simulink model "Car_22_Jan_test_2012b"  (R2012b)
settings: Solver=ode5  StartTime=0.0  StopTime=inf  FixedStep=sample_time  RelTol=1e-3
InitFcn:
  | sample_time=0.005;%0.004;%0.0025;%0.02;
  | sample_time_Vicon = 0.005;
  | DeltaT = 0.02;
  | g = 9.81;
  | H0 = g%0.3165;
  | Kl = 1;
  | 
  | Q6_mass = 0.84;
  | 
  | Q6_Omega_r = 1.5; %for horizon ref
  | Q6_Zeta_r = 0.5; %for horizon ref
  | Q6_Omega_r_h = 2;%for vertical ref
  | Q6_Zeta_r_h = 2; %for vertical ref
  | 
  | 
  | Q6_Omega = 1.5; %for horizon control
  | Q6_Zeta = 0.5; %for horizon control
  | Q6_Omega_h= 2; %for vertical control
  | Q6_Zeta_h = 0.7; %for vertical control
  | 
  | 
  | Q6_acc_max = 5;%horizontal max acc
  | Q6_acc_max_h = 3;%horizontal max acc
  | 
  | omega_circle = 72*pi/180;
  | omega_h = 0.1;%Ascending speed
  | PI = pi;
  | Circle_R = 2.5;
  | MAX_Height = -2;
undefined symbols (not defined in the file or in its folder): DiscIntNeverNeededParam
libraries: X330_Control x5, dspswit3 x5, simulink x4
(part 1 of 2)
settings Model: Creator=ttcl3  LastModifiedBy=Vicon
settings SolverCC: MaxConsecutiveMinStep=auto
settings DataIOCC: SignalLoggingSaveFormat=ModelDataLogs
settings DebuggingCC: MultiTaskRateTransMsg=warning  FcnCallInpInsideContextMsg=EnableAllAsWarning
settings SFSimCC: SimParseCustomCode=off
settings CodeAppCC: CustomSymbolStrType=$N$R$M_T
settings GRTTargetCC: CombineOutputUpdateFcns=off  GRTInterface=on

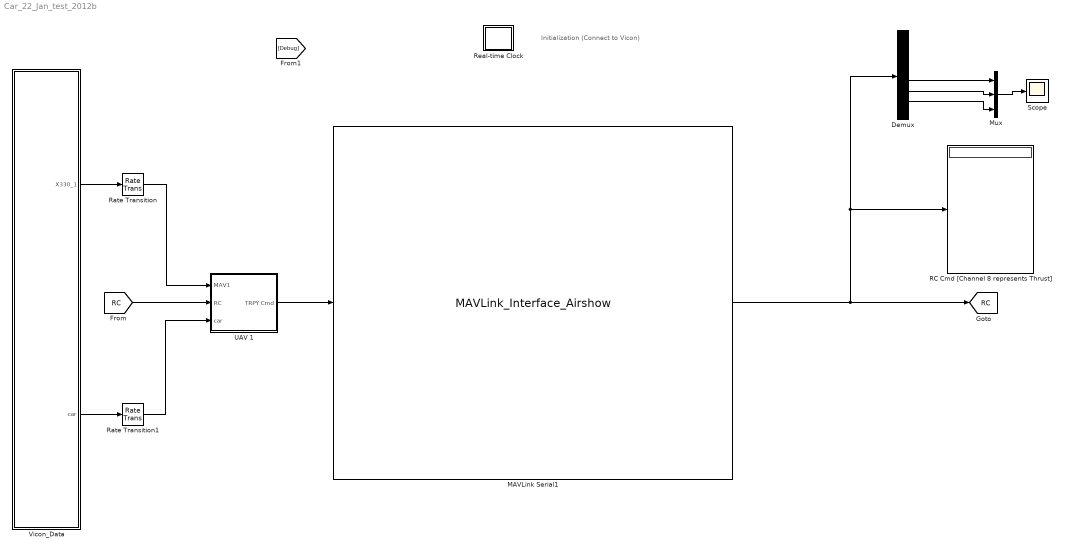
== system Car_22_Jan_test_2012b ==
  note: Initialization
      | (Connect to Vicon)
  Demux : Demux  Outputs=8
  MAVLink Serial1 : S-Function  FunctionName=MAVLink_Interface_Airshow  Parameters=COM_Port,Baud_Rate,MSG_INPUT,MSG_OUTPUT  EnableBusSupport=off  mask{COM_Port='COM5', Baud_Rate=57600, ATTITUDE_OUT=off, RC_SCALED=on, Quads_1=on, Quads_2=off, Quads_3=off, Quads_4=off, Quads_5=off, Quads_6=off}
      mask prompts: COM_Port "COM Port"; Baud_Rate "Baud Rate"; ATTITUDE_OUT "DEBUG"; RC_SCALED "RC CHANNELS SCALED"; Quads_1 "1 Quad"; Quads_2 "2 Quad"; Quads_3 "3 Quad"; Quads_4 "4 Quad"; Quads_5 "5 Quad"; Quads_6 "6 Quad"
      mask init:
      | MSG_ID_NUM_INPUT = [ uint8(221) uint8(222) uint8(223) uint8(224) uint8(225) uint8(226)];
      | MSG_ID_NAME_INPUT = [Quads_1 Quads_2 Quads_3 Quads_4 Quads_5 Quads_6];
      | 
      | MSG_ID_NUM_OUTPUT = [uint8(34) uint8(30)];
      | MSG_ID_NAME_OUTPUT = [RC_SCALED ATTITUDE_OUT ];
      | 
      | idx_input = find(MSG_ID_NAME_INPUT);
      | MSG_INPUT = MSG_ID_NUM_INPUT(idx_input);
      | 
      | idx_output = find(MSG_ID_NAME_OUTPUT);
      | MSG_OUTPUT = MSG_ID_NUM_OUTPUT(idx_output);
      mask Display:
      | % Block image
      | image(imread('10-inch Quad Heat Map.png'));
      | 
      | %Label block
      | fprintf('MAVLink Serial\n%s\n%dbps', COM_Port,  Baud_Rate)
      | 
      | 
      | %Label input ports
      | 
      | in = 1;
      | if (Quads_1 == 1)
      |     port_label('input', in, 'Quads_1');
      |     in = in + 1;
      | end
      | 
      | if (Quads_2 == 1)
      |     port_label('input', in, 'Quads_2');
      |     in = in + 1;
      | end
      | 
      | if (Quads_3 == 1)
      |     port_label('input', in, 'Quads_3');
      |     in = in + 1;
      | end
      | 
      | if (Quads_4 == 1)
      |     port_label('input', in, 'Quads_4');
      |     in = in + 1;
      | end
      | 
      | if (Quads_5 == 1)
      |     port_label('input', in, 'Quads_5');
      |     in = in + 1;
      | end
      | 
      | 
      | if (Quads_6 == 1)
      |     port_label('input', in, 'Quads_6');
      |     in = in + 1;
      | end
      | %Label output ports
      | 
      | out = 1;
      | if (RC_SCALED == 1)
      |     port_label('output', out, 'RC CMD');
      |     out = out + 1;
      | end
      | 
      | if (ATTITUDE_OUT == 1)
      |     port_label('output', out, 'DEBUG');
      |     out = out + 1;
      | end
  Mux : Mux  Inputs=3
  RC Cmd [Channel 8 represents Thrust] : Display
  Rate Transition : RateTransition  OutPortSampleTime=0.02
  Rate Transition1 : RateTransition  OutPortSampleTime=0.02
  Real-time Clock : Subsystem  mask(Real-time Clock){sample_time=0.02, tolerance=1}
      mask prompts: sample_time "Synchronize with real-time every n seconds:"; tolerance "Real-time warning tolerance (seconds):"
      mask help: Real-time Synchronization Block
      mask Help: This block synchronizes simulation time with the PC real-time clock or UNIX system clock. The first dialog entry is the period at which the clock is checked to insure real-time synchronization. The second dialog entry is the number of seconds that the simulation time must be within real-time before a warning is printed.
      mask Display: plot(0,0,100,100,[40,60,60,54,54,64,69,76,82,77,81,83,83,81,78,74,70,64,57,49,41,35,32,30,30,31,34,40,47,47,40,40],[90,90,85,85,80,79,76,87,80,70,64,57,49,41,33,28,24,22,21,23,25,31,37,46,56,65,73,78,80,85,85,90],[69,53,53],[64,50,73])
  Scope : Scope
  UAV 1 : Subsystem
  Vicon_Data : Subsystem
  tag scope: RC=global
  wires:
  [RC] -> UAV 1/2(RC)
  Vicon_Data/1(X330_1) -> Rate Transition/1
  Rate Transition/1 -> UAV 1/1(MAV1)
  UAV 1/1(TRPY Cmd) -> MAVLink Serial1/1
  Vicon_Data/2(car) -> Rate Transition1/1
  MAVLink Serial1/1 -> [RC], Demux/1, RC Cmd [Channel 8 represents Thrust]/1
  Rate Transition1/1 -> UAV 1/3(car)
  Demux/5 -> Mux/1
  Demux/6 -> Mux/2
  Demux/7 -> Mux/3
  Mux/1 -> Scope/1

== system Car_22_Jan_test_2012b/Real-time Clock ==
  Real-time Clock : S-Function  FunctionName=rtclock  Parameters=sample_time, tolerance  EnableBusSupport=off

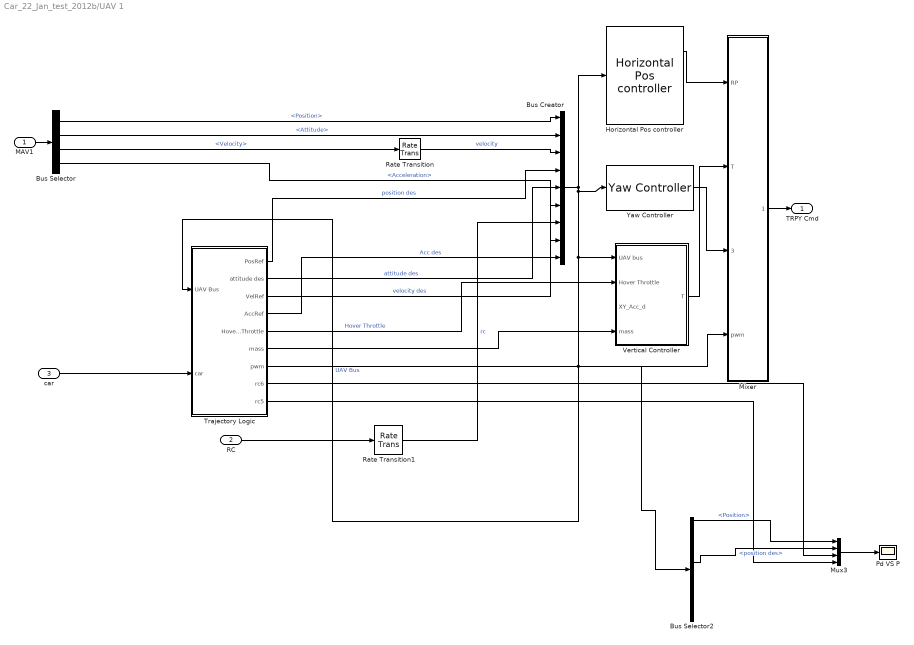
== system Car_22_Jan_test_2012b/UAV 1 ==
  MAV1 : Inport
  RC : Inport  Port=2
  car : Inport  Port=3
  Bus Creator : BusCreator  Inputs=9
  Bus Selector : BusSelector  OutputSignals=Position,Attitude,Velocity,Acceleration
  Bus Selector2 : BusSelector  OutputSignals=Position,Attitude,velocity,position des,attitude des,velocity des,rc,Acc des
  Horizontal Pos controller : X330_Control/Horizontal Pos controller  Max_RP=60  Omega=Q6_Omega  PID_i=1  Zeta=Q6_Zeta
  Mixer : Subsystem
  Mux3 : Mux
  Pd VS P : Scope
      settings: TimeRange=10  YMin=-1.5  YMax=2.25
  Rate Transition : RateTransition  OutPortSampleTime=0.02
  Rate Transition1 : RateTransition  OutPortSampleTime=0.02
  Trajectory Logic : Subsystem
  Vertical Controller : Subsystem  AncestorBlock=X330_Control/Vertical Controller  mask{Omega_h=Q6_Omega_h, Zeta_h=Q6_Zeta_h, PID_I_h=1, mass=Q6_mass}
      mask prompts: Omega_h "Omega (P Gain  = Omega^2)"; Zeta_h "Zeta (D Gain = 2*Omega*Zeta)"; PID_I_h "I Gain"
  Yaw Controller : X330_Control/Yaw Controller
  TRPY Cmd : Outport
  wires:
  Mux3/1 -> Pd VS P/1
  Bus Selector2/4 -> Mux3/2  "<position des>"
  Bus Selector2/1 -> Mux3/1  "<Position>"
  RC/1 -> Rate Transition1/1
  Trajectory Logic/4(AccRef) -> Bus Creator/9  "Acc des"
  Mixer/1(XYZ RPY) -> TRPY Cmd/1
  MAV1/1 -> Bus Selector/1
  Bus Selector/3 -> Rate Transition/1  "<Velocity>"
  Bus Selector/2 -> Bus Creator/2  "<Attitude>"
  Bus Selector/1 -> Bus Creator/1  "<Position>"
  Trajectory Logic/5(HoverThrottle) -> Vertical Controller/2(Hover Throttle)  "Hover Throttle"
  Trajectory Logic/3(VelRef) -> Bus Creator/6  "velocity des"
  Trajectory Logic/2(attitude des) -> Bus Creator/5  "attitude des"
  Trajectory Logic/1(PosRef) -> Bus Creator/4  "position des"
  Bus Selector/4 -> Bus Creator/8  "<Acceleration>"
  Vertical Controller/1(T) -> Mixer/2(T)
  Yaw Controller/1 -> Mixer/3(Yaw rate)
  Bus Creator/1 -> Yaw Controller/1, Bus Selector2/1, Trajectory Logic/1(UAV Bus), Vertical Controller/1(UAV bus), Horizontal Pos controller/1  "UAV Bus"
  Rate Transition1/1 -> Bus Creator/7  "rc"
  Rate Transition/1 -> Bus Creator/3  "velocity"
  Horizontal Pos controller/1 -> Mixer/1(RP)
  car/1 -> Trajectory Logic/2(car)
  Trajectory Logic/6(mass) -> Vertical Controller/4(mass)
  Trajectory Logic/7(pwm) -> Mixer/4(pwm)
  Trajectory Logic/8(rc6) -> Mux3/3
  Trajectory Logic/9(rc5) -> Mux3/4

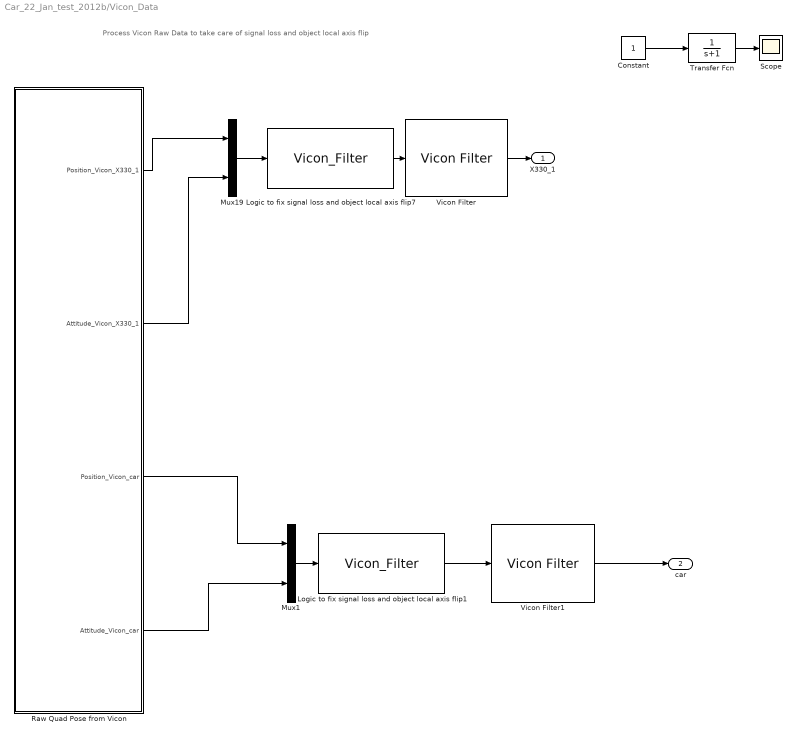
== system Car_22_Jan_test_2012b/Vicon_Data ==
  note: Process Vicon Raw Data to take care of signal loss and object local axis flip
  Constant : Constant  SampleTime=5
  Logic to fix signal loss and object local axis flip1 : M-S-Function  FunctionName=Vicon_Filter
  Logic to fix signal loss and object local axis flip7 : M-S-Function  FunctionName=Vicon_Filter
  Mux1 : Mux  Inputs=2
  Mux19 : Mux  Inputs=2
  Raw Quad Pose from Vicon : Subsystem
  Scope : Scope
      settings: SaveName=ScopeData2
  Transfer Fcn : TransferFcn  Denominator=[1 1]
  Vicon Filter : X330_Control/Vicon Filter
  Vicon Filter1 : X330_Control/Vicon Filter
  X330_1 : Outport
  car : Outport  Port=2
  wires:
  Mux19/1 -> Logic to fix signal loss and object local axis flip7/1
  Raw Quad Pose from Vicon/1(Position_Vicon_X330_1) -> Mux19/1
  Raw Quad Pose from Vicon/2(Attitude_Vicon_X330_1) -> Mux19/2
  Logic to fix signal loss and object local axis flip7/1 -> Vicon Filter/1
  Constant/1 -> Transfer Fcn/1
  Transfer Fcn/1 -> Scope/1
  Mux1/1 -> Logic to fix signal loss and object local axis flip1/1
  Logic to fix signal loss and object local axis flip1/1 -> Vicon Filter1/1
  Raw Quad Pose from Vicon/3(Position_Vicon_car) -> Mux1/1
  Raw Quad Pose from Vicon/4(Attitude_Vicon_car) -> Mux1/2
  Vicon Filter/1 -> X330_1/1
  Vicon Filter1/1 -> car/1

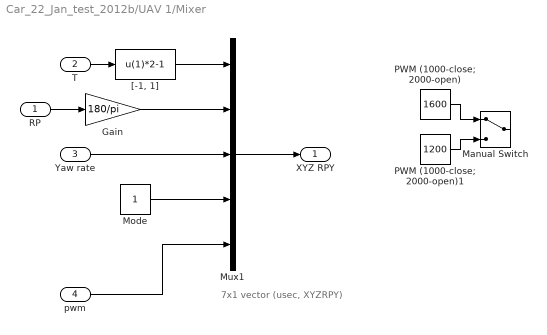
== system Car_22_Jan_test_2012b/UAV 1/Mixer ==
  note: 7x1 vector (usec, XYZRPY)
  RP : Inport
  T : Inport  Port=2
  Yaw rate : Inport  Port=3
  pwm : Inport  Port=4
  Gain : Gain  Gain=180/pi
  Manual Switch : ManualSwitch
  Mode : Constant  SampleTime=0.02
  Mux1 : Mux  Inputs=5
  PWM (1000-close; 2000-open) : Constant  Value=1600  SampleTime=0.02
  PWM (1000-close; 2000-open)1 : Constant  Value=1200  SampleTime=0.02
  "[-1, 1]" : Fcn  Expr=u(1)*2-1
  XYZ RPY : Outport
  wires:
  "[-1, 1]"/1 -> Mux1/1
  Gain/1 -> Mux1/2
  PWM (1000-close; 2000-open)1/1 -> Manual Switch/2
  PWM (1000-close; 2000-open)/1 -> Manual Switch/1
  Yaw rate/1 -> Mux1/3
  RP/1 -> Gain/1
  T/1 -> "[-1, 1]"/1
  Mux1/1 -> XYZ RPY/1
  Mode/1 -> Mux1/4
  pwm/1 -> Mux1/5

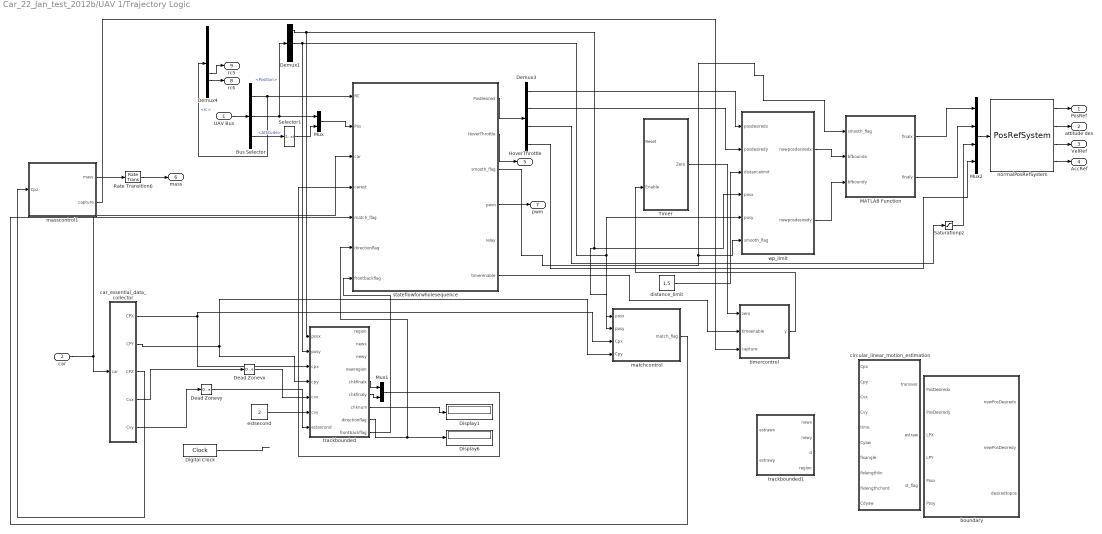
== system Car_22_Jan_test_2012b/UAV 1/Trajectory Logic ==
  UAV Bus : Inport
  car : Inport  Port=2
  Bus Selector : BusSelector  OutputSignals=rc,Position,Attitude
  Dead Zonevx : DeadZone  LowerValue=-0.1  UpperValue=0.1  SaturateOnIntegerOverflow=on
  Dead Zonevy : DeadZone  LowerValue=-0.1  UpperValue=0.1  SaturateOnIntegerOverflow=on
  Demux1 : Demux  Outputs=3
  Demux3 : Demux
  Demux4 : Demux  Outputs=8
  Digital Clock : DigitalClock  SampleTime=DeltaT
  Display1 : Display
  Display6 : Display
  MATLAB Function : MATLAB Function  TreatAsAtomicUnit=on
  Mux : Mux  Inputs=2
  Mux1 : Mux  Inputs=2
  Mux2 : Mux
  Rate Transition6 : RateTransition  OutPortSampleTime=0.02
  Saturationpz : Saturate  UpperLimit=0  LowerLimit=-2.5
  Selector1 : Selector  InputPortWidth=3  IndexOptions=Index vector (dialog)  Indices=[3]  OutputSizes=1
  Timer : Subsystem
  boundary : MATLAB Function  TreatAsAtomicUnit=on
  car_essential_data_collector : Subsystem
  circular_linear_motion_estimation : MATLAB Function  TreatAsAtomicUnit=on
  distance_limit : Constant  Value=1.5
  estsecond : Constant  Value=2
  masscontrol1 : MATLAB Function  TreatAsAtomicUnit=on
  matchcontrol : MATLAB Function  TreatAsAtomicUnit=on
  normalPosRefSystem : X330_Control/PosRefSystem  Omega_r=Q6_Omega_r  Zeta_r=Q6_Zeta_r  Acc_Max=Q6_acc_max  Omega_h_r=Q6_Omega_r_h  Zeta_h_r=Q6_Zeta_r_h  Acc_h_Max=Q6_acc_max_h
  stateflowforwholesequence : Stateflow chart  TreatAsAtomicUnit=on
  timercontrol : MATLAB Function  TreatAsAtomicUnit=on
  trackbounded : MATLAB Function  TreatAsAtomicUnit=on
  trackbounded1 : MATLAB Function  TreatAsAtomicUnit=on
  wp_limit : MATLAB Function  TreatAsAtomicUnit=on
  PosRef : Outport
  attitude des : Outport  Port=2
  VelRef : Outport  Port=3
  AccRef : Outport  Port=4
  HoverThrottle : Outport  Port=5
  mass : Outport  Port=6
  pwm : Outport  Port=7
  rc6 : Outport  Port=8
  rc5 : Outport  Port=9
  wires:
  Mux/1 -> stateflowforwholesequence/2(Pos)
  Selector1/1 -> Mux/2
  Bus Selector/3 -> Selector1/1  "<Attitude>"
  Bus Selector/2 -> Demux1/1, Mux/1  "<Position>"
  UAV Bus/1 -> Bus Selector/1
  stateflowforwholesequence/2(HoverThrottle) -> HoverThrottle/1
  Bus Selector/1 -> Demux4/1, stateflowforwholesequence/1(RC)  "<rc>"
  normalPosRefSystem/3 -> VelRef/1
  normalPosRefSystem/1 -> PosRef/1
  normalPosRefSystem/4 -> AccRef/1
  normalPosRefSystem/2 -> attitude des/1
  stateflowforwholesequence/1(PosDesired) -> Demux3/1
  Saturationpz/1 -> Mux2/3
  Mux2/1 -> normalPosRefSystem/1
  car/1 -> stateflowforwholesequence/3(car), car_essential_data_collector/1(car)
  car_essential_data_collector/1(CPX) -> trackbounded/3(cpx), matchcontrol/3(Cpx)
  car_essential_data_collector/2(CPY) -> trackbounded/4(cpy), matchcontrol/4(Cpy)
  Digital Clock/1 -> ?
  Dead Zonevx/1 -> trackbounded/5(cvx)
  Dead Zonevy/1 -> trackbounded/6(cvy)
  Demux3/1 -> wp_limit/1(posdesiredx)
  Demux3/2 -> wp_limit/2(posdesiredy)
  Demux3/3 -> Saturationpz/1
  Demux3/4 -> Mux2/4
  Demux1/1 -> matchcontrol/1(posx), wp_limit/4(posx), trackbounded/1(posx)
  Demux1/2 -> matchcontrol/2(posy), wp_limit/5(posy), trackbounded/2(posy)
  distance_limit/1 -> wp_limit/3(distancelimit)
  masscontrol1/1(mass) -> Rate Transition6/1
  stateflowforwholesequence/3(smooth_flag) -> MATLAB Function/1(smooth_flag), wp_limit/6(smooth_flag)
  car_essential_data_collector/3(CPZ) -> masscontrol1/1(Cpz)
  wp_limit/1(newposdesiredx) -> MATLAB Function/2(bfboundx)
  wp_limit/2(newposdesiredy) -> MATLAB Function/3(bfboundy)
  MATLAB Function/1(finalx) -> Mux2/1
  MATLAB Function/2(finaly) -> Mux2/2
  matchcontrol/1(match_flag) -> stateflowforwholesequence/5(match_flag)
  Rate Transition6/1 -> mass/1
  stateflowforwholesequence/4(pwm) -> pwm/1
  car_essential_data_collector/4(Cvx) -> Dead Zonevx/1
  car_essential_data_collector/5(Cvy) -> Dead Zonevy/1
  Demux4/7 -> rc6/1
  timercontrol/1(y) -> Timer/2(Enable)
  stateflowforwholesequence/6(timerenable) -> timercontrol/2(timeenable)
  Timer/1(Zero) -> timercontrol/1(zero)
  masscontrol1/2(capture) -> timercontrol/3(capture)
  Demux4/6 -> rc5/1
  estsecond/1 -> trackbounded/7(estsecond)
  trackbounded/7(chknum) -> Display1/1
  trackbounded/8(directionflag) -> stateflowforwholesequence/6(directionflag), Display6/1
  trackbounded/5(chkfinalx) -> Mux1/1
  trackbounded/6(chkfinaly) -> Mux1/2
  Mux1/1 -> stateflowforwholesequence/4(carest)
  trackbounded/9(frontbackflag) -> stateflowforwholesequence/7(frontbackflag)

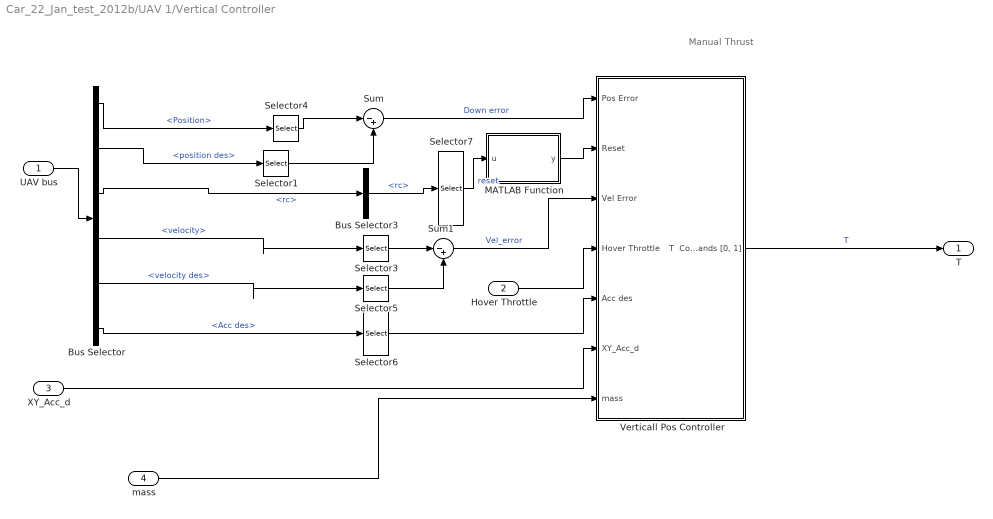
== system Car_22_Jan_test_2012b/UAV 1/Vertical Controller ==
  note: Manual Thrust
  UAV bus : Inport
  Hover Throttle : Inport  Port=2
  XY_Acc_d : Inport  Port=3
  mass : Inport  Port=4
  Bus Selector : BusSelector  OutputSignals=Position,position des,rc,velocity,velocity des,Acc des
  Bus Selector3 : BusSelector  OutputSignals=rc
  MATLAB Function : MATLAB Function  TreatAsAtomicUnit=on
  Selector{1,3..5} (4 alike) : Selector  InputPortWidth=3  IndexOptions=Index vector (dialog)  Indices=[3]  OutputSizes=1
  Selector6 : Selector  InputPortWidth=4  IndexOptions=Index vector (dialog)  Indices=[3]  OutputSizes=1
  Selector7 : Selector  InputPortWidth=8  IndexOptions=Index vector (dialog)  Indices=[7]  OutputSizes=1
  Sum : Sum  Inputs=|-+
  Sum1 : Sum  Inputs=|-+
  Verticall Pos Controller : Subsystem
  T : Outport
  wires:
  XY_Acc_d/1 -> Verticall Pos Controller/6(XY_Acc_d)
  Verticall Pos Controller/1("T  Commands [0, 1]") -> T/1  "T"
  Selector6/1 -> Verticall Pos Controller/5(Acc des)
  Bus Selector/6 -> Selector6/1  "<Acc des>"
  Hover Throttle/1 -> Verticall Pos Controller/4(Hover Throttle)
  Bus Selector/5 -> Selector5/1  "<velocity des>"
  Bus Selector/4 -> Selector3/1  "<velocity>"
  Selector5/1 -> Sum1/2
  Selector3/1 -> Sum1/1
  Sum1/1 -> Verticall Pos Controller/3(Vel Error)  "Vel_error"
  Selector7/1 -> MATLAB Function/1(u)  "reset"
  Bus Selector3/1 -> Selector7/1  "<rc>"
  Selector1/1 -> Sum/2
  Selector4/1 -> Sum/1
  Sum/1 -> Verticall Pos Controller/1(Pos Error)  "Down error"
  Bus Selector/2 -> Selector1/1  "<position des>"
  Bus Selector/1 -> Selector4/1  "<Position>"
  Bus Selector/3 -> Bus Selector3/1  "<rc>"
  UAV bus/1 -> Bus Selector/1
  mass/1 -> Verticall Pos Controller/7(mass)
  MATLAB Function/1(y) -> Verticall Pos Controller/2(Reset)

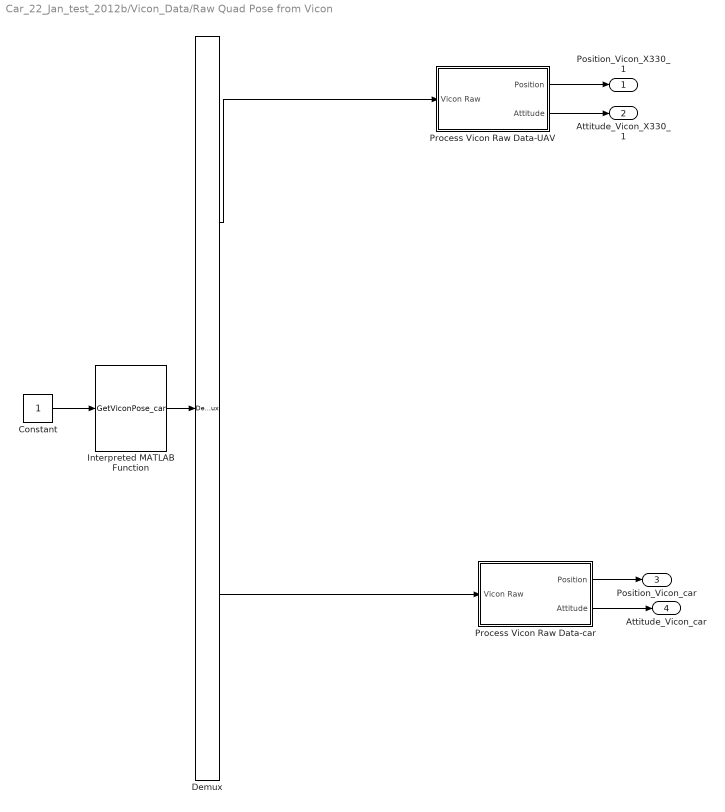
== system Car_22_Jan_test_2012b/Vicon_Data/Raw Quad Pose from Vicon ==
  Constant : Constant  SampleTime=sample_time
  Demux : Demux  Outputs=2
  Interpreted MATLAB Function : MATLABFcn  MATLABFcn=GetViconPose_car  OutputDimensions=12
  Process Vicon Raw Data-UAV : Subsystem
  Process Vicon Raw Data-car : Subsystem
  Position_Vicon_X330_1 : Outport
  Attitude_Vicon_X330_1 : Outport  Port=2
  Position_Vicon_car : Outport  Port=3
  Attitude_Vicon_car : Outport  Port=4
  wires:
  Interpreted MATLAB Function/1 -> Demux/1
  Process Vicon Raw Data-UAV/2(Attitude) -> Attitude_Vicon_X330_1/1
  Process Vicon Raw Data-UAV/1(Position) -> Position_Vicon_X330_1/1
  Demux/1 -> Process Vicon Raw Data-UAV/1(Vicon Raw)
  Constant/1 -> Interpreted MATLAB Function/1
  Process Vicon Raw Data-car/2(Attitude) -> Attitude_Vicon_car/1
  Process Vicon Raw Data-car/1(Position) -> Position_Vicon_car/1
  Demux/2 -> Process Vicon Raw Data-car/1(Vicon Raw)

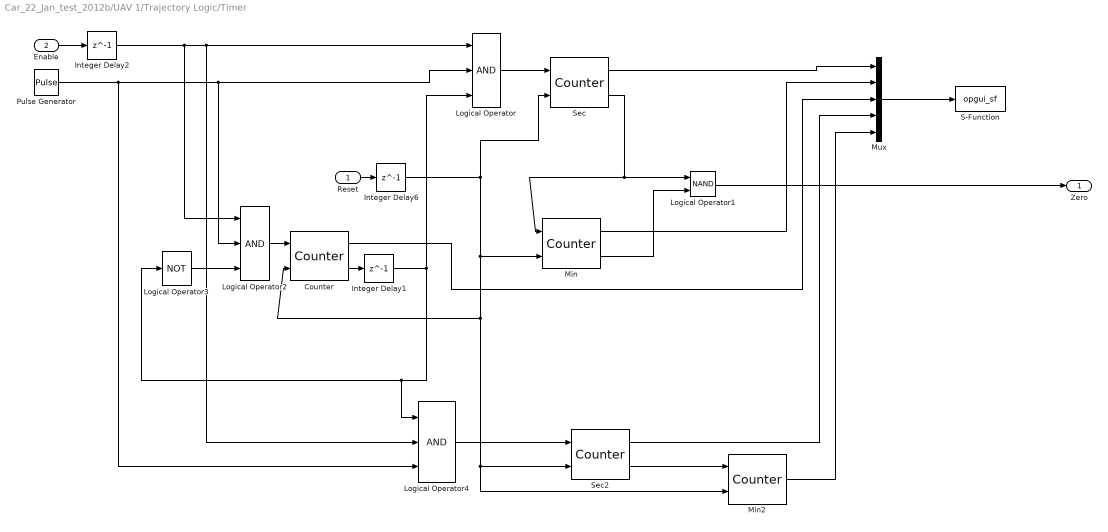
== system Car_22_Jan_test_2012b/UAV 1/Trajectory Logic/Timer ==
  Reset : Inport
  Enable : Inport  Port=2
  Counter : dspswit3/Counter  Direction=Down  CountEvent=Rising edge  CounterSize=User defined  MaxCount=4  InitialCount=4  Output=Count and Hit  HitValue=0  ResetInput=on  SamplesPerFrame=1  Ts=1  CntDtype=double  HitDtype=Boolean
  Integer Delay1 : Delay  DelayLength=1
  Integer Delay2 : Delay  DelayLength=1
  Integer Delay6 : Delay  DelayLength=1
  Logical Operator : Logic  Inputs=3  AllPortsSameDT=off  OutDataTypeStr=boolean
  Logical Operator1 : Logic  Operator=NAND  AllPortsSameDT=off  OutDataTypeStr=boolean
  Logical Operator2 : Logic  Inputs=3  AllPortsSameDT=off  OutDataTypeStr=boolean
  Logical Operator3 : Logic  Operator=NOT  Inputs=1  AllPortsSameDT=off  OutDataTypeStr=boolean
  Logical Operator4 : Logic  Inputs=3  AllPortsSameDT=off  OutDataTypeStr=boolean
  Min : dspswit3/Counter  Direction=Down  CountEvent=Rising edge  CounterSize=User defined  MaxCount=1  InitialCount=1  Output=Count and Hit  HitValue=0  ResetInput=on  SamplesPerFrame=1  Ts=1  CntDtype=double  HitDtype=Logical
  Min2 : dspswit3/Counter  Direction=Up  CountEvent=Rising edge  CounterSize=User defined  MaxCount=59  InitialCount=0  Output=Count  HitValue=0  ResetInput=on  SamplesPerFrame=1  Ts=1  CntDtype=double  HitDtype=Logical
  Mux : Mux  Inputs=5
  Pulse Generator : DiscretePulseGenerator  SampleTime=0.5
  S-Function : S-Function  FunctionName=opgui_sf  Parameters=0.5  EnableBusSupport=off
  Sec : dspswit3/Counter  Direction=Down  CountEvent=Rising edge  CounterSize=User defined  MaxCount=59  InitialCount=30  Output=Count and Hit  HitValue=0  ResetInput=on  SamplesPerFrame=1  Ts=1  CntDtype=double  HitDtype=Logical
  Sec2 : dspswit3/Counter  Direction=Up  CountEvent=Rising edge  CounterSize=User defined  MaxCount=59  InitialCount=0  Output=Count and Hit  HitValue=0  ResetInput=on  SamplesPerFrame=1  Ts=1  CntDtype=double  HitDtype=Logical
  Zero : Outport
  wires:
  Sec/2 -> Min/1, Logical Operator1/1
  Min/2 -> Logical Operator1/2
  Mux/1 -> S-Function/1
  Sec/1 -> Mux/1
  Logical Operator/1 -> Sec/1
  Counter/2 -> Integer Delay1/1
  Counter/1 -> Mux/3
  Min/1 -> Mux/2
  Logical Operator2/1 -> Counter/1
  Logical Operator3/1 -> Logical Operator2/3
  Enable/1 -> Integer Delay2/1
  Sec2/2 -> Min2/1
  Logical Operator4/1 -> Sec2/1
  Sec2/1 -> Mux/4
  Min2/1 -> Mux/5
  Integer Delay2/1 -> Logical Operator4/2, Logical Operator/1, Logical Operator2/1
  Pulse Generator/1 -> Logical Operator4/3, Logical Operator/2, Logical Operator2/2
  Reset/1 -> Integer Delay6/1
  Logical Operator1/1 -> Zero/1
  Integer Delay6/1 -> Sec/2, Counter/2, Sec2/2, Min2/2, Min/2
  Integer Delay1/1 -> Logical Operator/3, Logical Operator3/1, Logical Operator4/1

== system Car_22_Jan_test_2012b/UAV 1/Trajectory Logic/car_essential_data_collector ==
  car : Inport
  Demux : Demux  Outputs=12
  CPX : Outport
  CPY : Outport  Port=2
  CPZ : Outport  Port=3
  Cvx : Outport  Port=4
  Cvy : Outport  Port=5
  wires:
  car/1 -> Demux/1
  Demux/1 -> CPX/1
  Demux/2 -> CPY/1
  Demux/3 -> CPZ/1
  Demux/7 -> Cvx/1
  Demux/8 -> Cvy/1

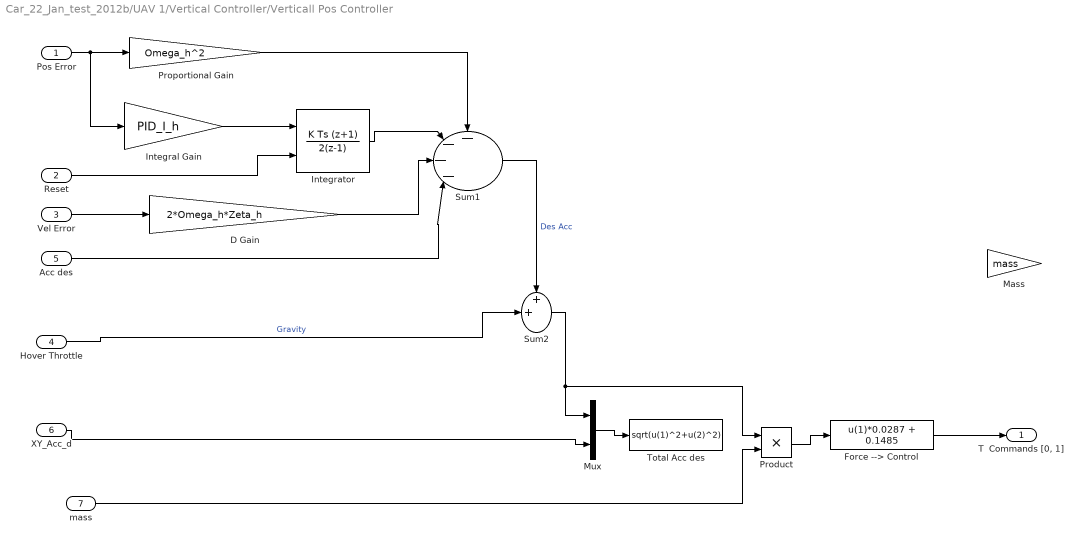
== system Car_22_Jan_test_2012b/UAV 1/Vertical Controller/Verticall Pos Controller ==
  Pos Error : Inport
  Reset : Inport  Port=2
  Vel Error : Inport  Port=3
  Hover Throttle : Inport  Port=4
  Acc des : Inport  Port=5
  XY_Acc_d : Inport  Port=6
  mass : Inport  Port=7
  D Gain : Gain  Gain=2*Omega_h*Zeta_h  OutDataTypeStr=double
  Force --> Control : Fcn  Expr=u(1)*0.0287 + 0.1485
  Integral Gain : Gain  DisableCoverage=on  Gain=PID_I_h  ParamDataTypeStr=double  OutDataTypeStr=double
  Integrator : DiscreteIntegrator  DisableCoverage=on  IntegratorMethod=Integration: Trapezoidal  ExternalReset=level  InitialConditionMode=State only (most efficient)  SampleTime=-1  OutDataTypeStr=double  UpperSaturationLimit=0.3  LowerSaturationLimit=-0.3  ICPrevOutput=DiscIntNeverNeededParam  ICPrevScaledInput=DiscIntNeverNeededParam
  Mass : Gain  DisableCoverage=on  Gain=mass  ParamDataTypeStr=double  OutDataTypeStr=double
  Mux : Mux  Inputs=2
  Product : Product  RndMeth=Zero
  Proportional Gain : Gain  DisableCoverage=on  Gain=Omega_h^2  ParamDataTypeStr=double  OutDataTypeStr=double
  Sum1 : Sum  DisableCoverage=on  Inputs=----|  AccumDataTypeStr=double  OutDataTypeStr=double  SampleTime=0.02
  Sum2 : Sum  DisableCoverage=on  Inputs=++|  AccumDataTypeStr=double  OutDataTypeStr=double  SampleTime=0.02
  Total Acc des : Fcn  Expr=sqrt(u(1)^2+u(2)^2)
  "T  Commands [0, 1]" : Outport
  wires:
  Force --> Control/1 -> "T  Commands [0, 1]"/1
  Sum2/1 -> Product/1, Mux/1
  XY_Acc_d/1 -> Mux/2
  Mux/1 -> Total Acc des/1
  Product/1 -> Force --> Control/1
  Sum1/1 -> Sum2/1  "Des Acc"
  Hover Throttle/1 -> Sum2/2  "Gravity"
  Acc des/1 -> Sum1/4
  D Gain/1 -> Sum1/3
  Vel Error/1 -> D Gain/1
  Reset/1 -> Integrator/2
  Pos Error/1 -> Integral Gain/1, Proportional Gain/1
  Proportional Gain/1 -> Sum1/1
  Integrator/1 -> Sum1/2
  Integral Gain/1 -> Integrator/1
  mass/1 -> Product/2

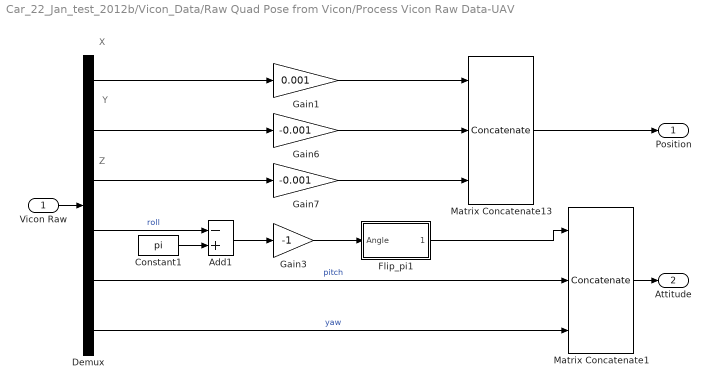
== system Car_22_Jan_test_2012b/Vicon_Data/Raw Quad Pose from Vicon/Process Vicon Raw Data-UAV ==
  note: X
  note: Y
  note: Z
  Vicon Raw : Inport
  Add1 : Sum  Inputs=-+
  Constant1 : Constant  Value=pi  OutDataTypeStr=double
  Demux : Demux  Outputs=6
  Flip_pi1 : Subsystem  mask(Flip -pi to pi){}
      mask help: Flips the inputs into the range -pi to pi
      mask Help: Flips the inputs into the range -pi to pi
      mask Display: disp('Flip_pi')
  Gain1 : Gain  Gain=0.001
  Gain3 : Gain  Gain=-1
  Gain6 : Gain  Gain=-0.001
  Gain7 : Gain  Gain=-0.001
  Matrix Concatenate1 : Concatenate  NumInputs=3  Mode=Multidimensional array
  Matrix Concatenate13 : Concatenate  NumInputs=3  Mode=Multidimensional array
  Position : Outport
  Attitude : Outport  Port=2
  wires:
  Constant1/1 -> Add1/2
  Demux/6 -> Matrix Concatenate1/3  "yaw"
  Gain1/1 -> Matrix Concatenate13/1
  Demux/1 -> Gain1/1
  Demux/2 -> Gain6/1
  Demux/3 -> Gain7/1
  Demux/4 -> Add1/1  "roll"
  Gain6/1 -> Matrix Concatenate13/2
  Gain7/1 -> Matrix Concatenate13/3
  Add1/1 -> Gain3/1
  Gain3/1 -> Flip_pi1/1(Angle)
  Demux/5 -> Matrix Concatenate1/2  "pitch"
  Flip_pi1/1(Angle_Flip) -> Matrix Concatenate1/1
  Matrix Concatenate13/1 -> Position/1
  Vicon Raw/1 -> Demux/1
  Matrix Concatenate1/1 -> Attitude/1

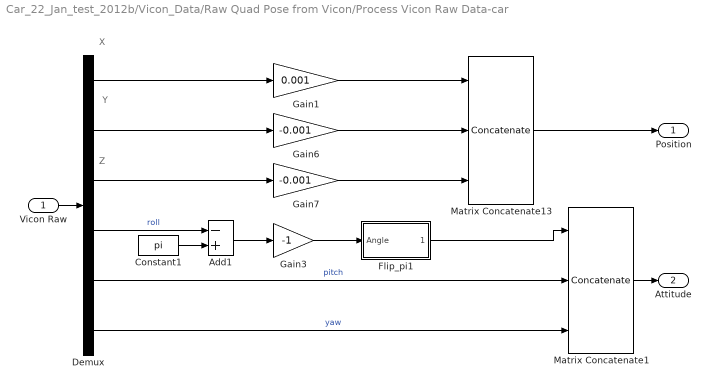
== system Car_22_Jan_test_2012b/Vicon_Data/Raw Quad Pose from Vicon/Process Vicon Raw Data-car ==
  note: X
  note: Y
  note: Z
  Vicon Raw : Inport
  Add1 : Sum  Inputs=-+
  Constant1 : Constant  Value=pi  OutDataTypeStr=double
  Demux : Demux  Outputs=6
  Flip_pi1 : Subsystem  mask(Flip -pi to pi){}
      mask help: Flips the inputs into the range -pi to pi
      mask Help: Flips the inputs into the range -pi to pi
      mask Display: disp('Flip_pi')
  Gain1 : Gain  Gain=0.001
  Gain3 : Gain  Gain=-1
  Gain6 : Gain  Gain=-0.001
  Gain7 : Gain  Gain=-0.001
  Matrix Concatenate1 : Concatenate  NumInputs=3  Mode=Multidimensional array
  Matrix Concatenate13 : Concatenate  NumInputs=3  Mode=Multidimensional array
  Position : Outport
  Attitude : Outport  Port=2
  wires:
  Constant1/1 -> Add1/2
  Demux/6 -> Matrix Concatenate1/3  "yaw"
  Gain1/1 -> Matrix Concatenate13/1
  Demux/1 -> Gain1/1
  Demux/2 -> Gain6/1
  Demux/3 -> Gain7/1
  Demux/4 -> Add1/1  "roll"
  Gain6/1 -> Matrix Concatenate13/2
  Gain7/1 -> Matrix Concatenate13/3
  Add1/1 -> Gain3/1
  Gain3/1 -> Flip_pi1/1(Angle)
  Demux/5 -> Matrix Concatenate1/2  "pitch"
  Flip_pi1/1(Angle_Flip) -> Matrix Concatenate1/1
  Matrix Concatenate13/1 -> Position/1
  Vicon Raw/1 -> Demux/1
  Matrix Concatenate1/1 -> Attitude/1

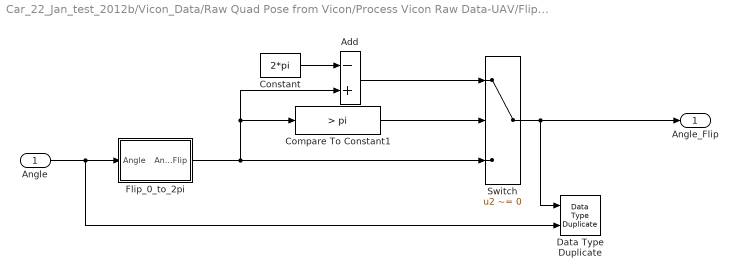
== system Car_22_Jan_test_2012b/Vicon_Data/Raw Quad Pose from Vicon/Process Vicon Raw Data-UAV/Flip_pi1 ==
  Angle : Inport
  Add : Sum  Inputs=-+
  Compare To Constant1 : simulink/Logic and Bit Operations/Compare To Constant  relop=>  const=pi  OutDataTypeStr=uint8  ZeroCross=off
  Constant : Constant  Value=2*pi
  Data Type Duplicate : DataTypeDuplicate
  Flip_0_to_2pi : Subsystem  mask(Flip zero to 2pi){}
      mask help: Flips the inputs into the range zero to +2pi
      mask Help: Flips the inputs into the range zero to +2pi
      mask Display: disp('Flip_0_2pi')
  Switch : Switch  Criteria=u2 ~= 0
  Angle_Flip : Outport
  wires:
  Switch/1 -> Data Type Duplicate/1, Angle_Flip/1
  Add/1 -> Switch/1
  Constant/1 -> Add/1
  Compare To Constant1/1 -> Switch/2
  Flip_0_to_2pi/1(Angle_Flip) -> Add/2, Compare To Constant1/1, Switch/3
  Angle/1 -> Data Type Duplicate/2, Flip_0_to_2pi/1(Angle)

== system Car_22_Jan_test_2012b/Vicon_Data/Raw Quad Pose from Vicon/Process Vicon Raw Data-car/Flip_pi1 ==
  Angle : Inport
  Add : Sum  Inputs=-+
  Compare To Constant1 : simulink/Logic and Bit Operations/Compare To Constant  relop=>  const=pi  OutDataTypeStr=uint8  ZeroCross=off
  Constant : Constant  Value=2*pi
  Data Type Duplicate : DataTypeDuplicate
  Flip_0_to_2pi : Subsystem  mask(Flip zero to 2pi){}
      mask help: Flips the inputs into the range zero to +2pi
      mask Help: Flips the inputs into the range zero to +2pi
      mask Display: disp('Flip_0_2pi')
  Switch : Switch  Criteria=u2 ~= 0
  Angle_Flip : Outport
  wires:
  Switch/1 -> Data Type Duplicate/1, Angle_Flip/1
  Add/1 -> Switch/1
  Constant/1 -> Add/1
  Compare To Constant1/1 -> Switch/2
  Flip_0_to_2pi/1(Angle_Flip) -> Add/2, Compare To Constant1/1, Switch/3
  Angle/1 -> Data Type Duplicate/2, Flip_0_to_2pi/1(Angle)

== system Car_22_Jan_test_2012b/Vicon_Data/Raw Quad Pose from Vicon/Process Vicon Raw Data-UAV/Flip_pi1/Flip_0_to_2pi ==
  Angle : Inport
  Add : Sum
  Compare To Constant1 : simulink/Logic and Bit Operations/Compare To Constant  relop=<  const=0  OutDataTypeStr=uint8  ZeroCross=off
  Constant : Constant  Value=2*pi
  Data Type Duplicate : DataTypeDuplicate
  Flip_2pi : Subsystem  mask(Flip -2pi to 2pi){}
      mask help: Flips the inputs into the range -2pi to +2pi
      mask Help: Flips the inputs into the range -2pi to +2pi
      mask Display: disp('Flip_2pi')
  Switch : Switch  Criteria=u2 ~= 0
  Angle_Flip : Outport
  wires:
  Switch/1 -> Data Type Duplicate/1, Angle_Flip/1
  Angle/1 -> Data Type Duplicate/2, Flip_2pi/1(Angle)
  Add/1 -> Switch/1
  Constant/1 -> Add/1
  Compare To Constant1/1 -> Switch/2
  Flip_2pi/1(Angle_Flip) -> Switch/3, Add/2, Compare To Constant1/1

== system Car_22_Jan_test_2012b/Vicon_Data/Raw Quad Pose from Vicon/Process Vicon Raw Data-car/Flip_pi1/Flip_0_to_2pi ==
  Angle : Inport
  Add : Sum
  Compare To Constant1 : simulink/Logic and Bit Operations/Compare To Constant  relop=<  const=0  OutDataTypeStr=uint8  ZeroCross=off
  Constant : Constant  Value=2*pi
  Data Type Duplicate : DataTypeDuplicate
  Flip_2pi : Subsystem  mask(Flip -2pi to 2pi){}
      mask help: Flips the inputs into the range -2pi to +2pi
      mask Help: Flips the inputs into the range -2pi to +2pi
      mask Display: disp('Flip_2pi')
  Switch : Switch  Criteria=u2 ~= 0
  Angle_Flip : Outport
  wires:
  Switch/1 -> Data Type Duplicate/1, Angle_Flip/1
  Angle/1 -> Data Type Duplicate/2, Flip_2pi/1(Angle)
  Add/1 -> Switch/1
  Constant/1 -> Add/1
  Compare To Constant1/1 -> Switch/2
  Flip_2pi/1(Angle_Flip) -> Switch/3, Add/2, Compare To Constant1/1

== system Car_22_Jan_test_2012b/Vicon_Data/Raw Quad Pose from Vicon/Process Vicon Raw Data-UAV/Flip_pi1/Flip_0_to_2pi/Flip_2pi ==
  Angle : Inport
  Bias : Bias  Bias=-2*pi
  Constant : Constant  Value=2*pi
  Data Type Duplicate : DataTypeDuplicate
  Modulo : Math  Operator=mod  SaturateOnIntegerOverflow=on
  Sign1 : Signum
  Switch : Switch
  Angle_Flip : Outport
  wires:
  Switch/1 -> Data Type Duplicate/2, Angle_Flip/1
  Bias/1 -> Switch/3
  Sign1/1 -> Switch/2
  Modulo/1 -> Switch/1, Bias/1
  Constant/1 -> Modulo/2
  Angle/1 -> Data Type Duplicate/1, Sign1/1, Modulo/1

== system Car_22_Jan_test_2012b/Vicon_Data/Raw Quad Pose from Vicon/Process Vicon Raw Data-car/Flip_pi1/Flip_0_to_2pi/Flip_2pi ==
  Angle : Inport
  Bias : Bias  Bias=-2*pi
  Constant : Constant  Value=2*pi
  Data Type Duplicate : DataTypeDuplicate
  Modulo : Math  Operator=mod  SaturateOnIntegerOverflow=on
  Sign1 : Signum
  Switch : Switch
  Angle_Flip : Outport
  wires:
  Switch/1 -> Data Type Duplicate/2, Angle_Flip/1
  Bias/1 -> Switch/3
  Sign1/1 -> Switch/2
  Modulo/1 -> Switch/1, Bias/1
  Constant/1 -> Modulo/2
  Angle/1 -> Data Type Duplicate/1, Sign1/1, Modulo/1

== matlab function Car_22_Jan_test_2012b/UAV 1/Trajectory Logic/circular_linear_motion_estimation ==
  data: Cpx input; Cpy input; Cvx input; Cvy input; transvec output; estraw output; st_flag output; time input; Cyaw input; fixangle input; fixlengthlin input; fixlengthchord input; Cdyaw input
function [transvec,estraw,st_flag] = fcn(Cpx,Cpy,Cvx,Cvy,time,Cyaw,fixangle,fixlengthlin,fixlengthchord,Cdyaw)
if(Cvx == 0 && Cvy == 0)
    st_flag = 1;
else 
    st_flag = 0;
end
%%%%%%%%%%%%%%%%%%%%%%circular estimation%%%%%%%%%%%%%%%%%%%%%%%%%%%%
%vxyM = sqrt((Cvx)^2 + (Cvy)^2); %resultant vector vxy
if(st_flag == 0)
    
        angleOmega = Cyaw + 0.5 * fixangle * pi / 180; %angleOmega(radian): between vx and L
        zero_chk = 1;
else
    
      angleOmega = 0;  
      zero_chk = 0;
end
if(Cdyaw ~= 0) %use dyaw to select circular or linear estimation
%r = vxyM / abs(Cdyaw);
%Chord = 2 * r * sin(fixangle * pi / 360); %%%%%chord sometime will go to
%very large value, will disable this parameter soon
transveccir = [fixlengthchord * cos(angleOmega)*zero_chk  fixlengthchord * sin(angleOmega) * zero_chk];
transveclin = [0 0];
else
%%%%%%%%%%%%%%%%%%%%%%%%linear estimation%%%%%%%%%%%%%%%%%%%%%%%%%%%%%%
transveclin = [fixlengthlin * cos(Cyaw * pi / 180)*zero_chk fixlengthlin * sin(Cyaw * pi / 180)*zero_chk];
transveccir = [0 0];
%Chord = 0;
end
if(time<2)       %%%%%%%%%%%%%%%%%avoid noise when initializing the program in first 2 seconds
    transvec = [0 0];
else
transvec = transveccir + transveclin;
end

C2dvec = [Cpx Cpy];
estraw = C2dvec + transvec;

== matlab function Car_22_Jan_test_2012b/UAV 1/Trajectory Logic/wp_limit ==
  data: posdesiredx input; posdesiredy input; distancelimit input; posx input; posy input; newposdesiredx output; newposdesiredy output; smooth_flag input
function [newposdesiredx,newposdesiredy] = fcn(posdesiredx,posdesiredy,distancelimit,posx,posy,smooth_flag)
%#codegen
w = atan2((posdesiredx-posx),(posdesiredy-posy));
desiredtopos = sqrt((posdesiredy-posy)^2+(posdesiredx-posx)^2);
if(smooth_flag == 1)
    newposdesiredx = posdesiredx;
    newposdesiredy = posdesiredy;
    %newposdesiredx = posx + smoothdistancelimit*sin(w);
    %newposdesiredy = posy + smoothdistancelimit*cos(w);
else
if(desiredtopos <= distancelimit)
    newposdesiredx = posdesiredx;
    newposdesiredy = posdesiredy;
else
    newposdesiredx = posx + distancelimit*sin(w);
    newposdesiredy = posy + distancelimit*cos(w);
end
end

== matlab function Car_22_Jan_test_2012b/UAV 1/Trajectory Logic/trackbounded1 ==
  data: newx output; newy output; estrawx input; estrawy input; d output; region output
function [newx,newy,d,region]  = fcn(estrawx,estrawy)
%#codegen
%cp = [cpy,cpx,0];
cpest = [estrawy, estrawx,0];
%%database of check points
chk0x = -0.4383;
chk0y = -0.9285;
chk1x = 1.047;
chk1y = -0.9693;
chk2x = 1.396;
chk2y = 0.4535;
chk3x = 1.382;
chk3y = 1.505;
chk4x = 1.042;
chk4y = 1.925;
chk5x = 0.3708;
chk5y = 1.821;
%%chk5x = ;
%%chk....
chk0 = [chk0y,chk0x,0];
chk1 = [chk1y,chk1x,0];
chk2 = [chk2y,chk2x,0];
chk3 = [chk3y,chk3x,0];
chk4 = [chk4y,chk4x,0];
chk5 = [chk5y,chk5x,0];
%%%%%%%%%%%%%%%%%%%%%%%%%%%%%%%%%%%%%%%%%%%%%%%%%%%%%%%%%%%%%%%%%%%%%%%%%%%%%%%%%%%%%%region selector
if(estrawx>2 && estrawx<=3 && estrawy>-3 && estrawy<=-2)
    region = 0;
elseif(estrawx>2 && estrawx<=3 && estrawy>-2 && estrawy<=-1 )
    region = 1;
elseif(estrawx>2 && estrawx<=3 && estrawy>-1 && estrawy<=0 )
    region = 2;
elseif(estrawx>2 && estrawx<=3 && estrawy>0 && estrawy<=1 )
    region = 3;
elseif(estrawx>2 && estrawx<=3 && estrawy>1 && estrawy<=2)
    region = 4;
elseif(estrawx>2 && estrawx<=3 && estrawy>2 && estrawy<=3)
    region = 5;
elseif(estrawx>1 && estrawx<=2 && estrawy>-3 && estrawy<=-2)
    region = 6;
elseif(estrawx>1 && estrawx<=2 && estrawy>-2 && estrawy<=-1)
    region = 7;
elseif(estrawx>1 && estrawx<=2 && estrawy>-1 && estrawy<=0)
    region = 8;
elseif(estrawx>1 && estrawx<=2 && estrawy>0 && estrawy<=1)
    region = 9;
elseif(estrawx>1 && estrawx<=2 && estrawy>1 && estrawy<=2)
    region = 10;
elseif(estrawx>1 && estrawx<=2 && estrawy>2 && estrawy<=3)
    region = 11;
elseif(estrawx>0 && estrawx<=1 && estrawy>-3 && estrawy<=-2)
    region = 12;
elseif(estrawx>0 && estrawx<=1 && estrawy>-2 && estrawy<=-1)
    region = 13;
elseif(estrawx>0 && estrawx<=1 && estrawy>-1 && estrawy<=0)
    region = 14;
elseif(estrawx>0 && estrawx<=1 && estrawy>0 && estrawy<=1)
    region = 15;
elseif(estrawx>0 && estrawx<=1 && estrawy>1 && estrawy<=2)
    region = 16;
elseif(estrawx>0 && estrawx<=1 && estrawy>2 && estrawy<=3)
    region = 17;
elseif(estrawx>-1 && estrawx<=0 && estrawy>-3 && estrawy<=-2)
    region = 18;
elseif(estrawx>-1 && estrawx<=0 && estrawy>-2 && estrawy<=-1)
    region = 19;
elseif(estrawx>-1 && estrawx<=0 && estrawy>-1 && estrawy<=0)
    region = 20;
elseif(estrawx>-1 && estrawx<=0 && estrawy>0 && estrawy<=1)
    region = 21;
elseif(estrawx>-1 && estrawx<=0 && estrawy>1 && estrawy<=2)
    region = 22;
elseif(estrawx>-1 && estrawx<=0 && estrawy>2 && estrawy<=3)
    region = 23;
elseif(estrawx>-2 && estrawx<=-1 && estrawy>-3 && estrawy<=-2)
    region = 24;
elseif(estrawx>-2 && estrawx<=-1 && estrawy>-2 && estrawy<=-1)
    region = 25;
elseif(estrawx>-2 && estrawx<=-1 && estrawy>-1 && estrawy<=0)
    region = 26;
elseif(estrawx>-2 && estrawx<=-1 && estrawy>0 && estrawy<=1)
    region = 27;
elseif(estrawx>-2 && estrawx<=-1 && estrawy>1 && estrawy<=2)
    region = 28;
elseif(estrawx>-2 && estrawx<=-1 && estrawy>2 && estrawy<=3)
    region = 29;
elseif(estrawx>-3 && estrawx<=-2 && estrawy>-3 && estrawy<=-2)
    region = 30;
elseif(estrawx>-3 && estrawx<=-2 && estrawy>-2 && estrawy<=-1)
    region = 31;
elseif(estrawx>-3 && estrawx<=-2 && estrawy>-1 && estrawy<=0)
    region = 32;
elseif(estrawx>-3 && estrawx<=-2 && estrawy>0 && estrawy<=1)
    region = 33;
elseif(estrawx>-3 && estrawx<=-2 && estrawy>1 && estrawy<=2)
    region = 34;
elseif(estrawx>-3 && estrawx<=-2 && estrawy>2 && estrawy<=3)
    region = 35;
else
    region = -1;
end
%%%%%%%%%%%%%%%%%%%%%%%%%%%%%%%%%%%%%%%%%%%%%%%%%%%%%%%%%%%%%%%%%%%%%%%%%%%%%%%%%%%%%%%%%%%%%%%%%%
if(region == 20 || region==19||region==13||region==14||region==7||region==21||region==6||region==12||region==18||region==24||region==25||region==26||region==27)
    %%%%%%%%%%%%%%%%calculate point to line distance%%%%%%%%%%%
    a = chk1 - chk0;
    b = cpest - chk0;
    d = norm(cross(a,b)) / norm(a);
    angle = atan2((chk1x-chk0x),(chk1y-chk0y));
    samplex = chk0x;
    sampley = chk0y;
    samplefinalx = chk1x;
    samplefinaly = chk1y;
    zero = 1;
elseif(region == 2||region==1||region==0||region==8)
    a = chk2 - chk1;
    b = cpest - chk1;
    d = norm(cross(a,b)) / norm(a);
    angle = atan2((chk2x-chk1x),(chk2y-chk1y));
    zero = 1;
    samplex = chk1x;
    sampley = chk1y;
    samplefinalx = chk2x;
    samplefinaly = chk2y;
elseif(region == 3||region==9||region==15)
    a = chk3 - chk2;
    b = cpest - chk2;
    d = norm(cross(a,b)) / norm(a);
    angle = atan2((chk3x-chk2x),(chk3y-chk2y));
    zero = 1;
    samplex = chk2x;
    sampley = chk2y;
    samplefinalx = chk3x;
    samplefinaly = chk3y;
elseif(region == 5||region==5||region==10||region==11)
    a = chk4 - chk3;
    b = cpest - chk3;
    d = norm(cross(a,b)) / norm(a);
    angle = atan2((chk4x-chk3x),(chk4y-chk3y));
    zero = 1;  
    samplex = chk3x;
    sampley = chk3y;
    samplefinalx = chk4x;
    samplefinaly = chk4y;
elseif(region == 16||region==17||region==22||region==23||region==28||region==29||region==34||region==35)
    a = chk5 - chk4;
    b = cpest - chk4;
    d = norm(cross(a,b)) / norm(a);
    angle = atan2((chk5x-chk4x),(chk5y-chk4y));
    zero = 1;
     samplex = chk4x;
    sampley = chk4y;
    samplefinalx = chk5x;
    samplefinaly = chk5y;

else
    a = -1;
    b = -1;
    d = -1;
    angle = -1;%%% i know this is not correct i will add one more zero coefficient to cancel this case
    zero = 0;
    samplex = 0;
    sampley = 0;
    samplefinalx = 0;
    samplefinaly = 0;
end
%%%%%%%%%%%%%%%%%%%%%%%%%%%%%%%%%%%%%%%%%%%%%%%%%%%%%%%%%%%%%%%%%%%%%%%%%%%%%%%%%%%%%%%%%%%%%%%%%%
%%calculate project point on the check point line
if(region == -1)%%if out of boundary none of the region match
        newy = 0;
        newx = 0;
else   %%match the region

distance = sqrt((samplefinalx-estrawx)^2+(samplefinaly-estrawy)^2); 
%if(distance > 1)
    %newx = samplefinalx;
   % newy = samplefinaly;
%else
      if(d<0.75)%%test the boundary width normal case if less than 0.75 m
    newx = estrawx;
    newy = estrawy;
      else%% out of boundary
        if(angle == 0 ||angle == 180)
            newx  = samplex;
            newy = estrawy;
        elseif(angle == 90 || angle == 270)
            newx = estrawx;
            newy = sampley;
        else
         kk = -1/(tan(angle));
         m = estrawx - kk*estrawy ;
         k = tan(angle);
         newy = (samplex - k*sampley - m)/(kk - k);
         newx = kk*newy + m;
        end
      end
%end
end

== matlab function Car_22_Jan_test_2012b/UAV 1/Trajectory Logic/boundary ==
  data: PosDesiredx input; newPosDesiredx output; PosDesiredy input; LPX input; LPY input; Posx input; Posy input; newPosDesiredy output; desiredtopos output
function [newPosDesiredx, newPosDesiredy,desiredtopos] = fcn(PosDesiredx,PosDesiredy, LPX,LPY,Posx,Posy)

UAVreal = [Posy, Posx,0];
UAVdesired = [PosDesiredy, PosDesiredx,0];
LA = [LPY, LPX,0];
r = 1.2;%%%%%landing_area circle radius
%%%%%%%%%%%%%%%%calculate point to line distance%%%%%%%%%%%
if(PosDesiredx == Posx && PosDesiredy == Posy)
    d = 1.3; %%%%%%%%%%%whatever value larger than 1.2, just for if this is not a line but a point
else
    a = UAVdesired - UAVreal;
    b = LA - UAVreal;
    d = norm(cross(a,b)) / norm(a);
end
%%%%%%%%%%%%%%%%%%%%%%%%%%%%%%%%%%%%%%%%%%%%%%%%%%%%%%%%%%
k = (PosDesiredx-Posx)/(PosDesiredy-Posy);
m = -k*PosDesiredy + PosDesiredx - LPX;
desiredtopos = sqrt((PosDesiredy-Posy)^2+(PosDesiredx-Posx)^2);
w = 0;
angleLAtoPos=atan2((Posx-LPX),(Posy-LPY));
if((Posx-LPX)^2+(Posy-LPY)^2<=r^2)%%%uav inside the circle already
    newPosDesiredx = LPX + r*cos(angleLAtoPos);
    newPosDesiredy = LPY + r*sin(angleLAtoPos);
else%%%%%%%uav outside the circle
if(d>=r)%%outside or tangent with circle
    n = 0;
    w = 0;
    zerochk = 0;
    wperpendicular = (w + 0.5 * pi)*zerochk;
    intersecty1 = Posy;
    intersecty2 = Posy;
    intersectx1 = Posx;
    intersectx2 = Posx;
    intersec1topos = sqrt((intersecty1-Posy)^2 + (intersectx1-Posx)^2);
    intersec2topos = sqrt((intersecty2-Posy)^2 + (intersectx2-Posx)^2);
    newPosDesiredy = PosDesiredy;
    newPosDesiredx = PosDesiredx;
else 
    n = sqrt(4*(LPY - k*m)^2 - 4*(k^2+1)*(LPY^2 + m^2 - r^2));
    intersecty1 = (2*(LPY - k*m)+n)/(2*(k^2+1));
    intersecty2 = (2*(LPY - k*m)-n)/(2*(k^2+1));
    intersectx1 = k*(intersecty1 - PosDesiredy)+PosDesiredx;
    intersectx2 = k*(intersecty2 - PosDesiredy)+PosDesiredx;
    intersec1topos = sqrt((intersecty1-Posy)^2 + (intersectx1-Posx)^2);
    intersec2topos = sqrt((intersecty2-Posy)^2 + (intersectx2-Posx)^2);
    if(intersec1topos<intersec2topos)
        w = atan2((LPX-intersectx1),(LPY-intersecty1));
    else
        w = atan2((LPX-intersectx2),(LPY-intersecty2));
    end
        if(desiredtopos<=intersec1topos && desiredtopos<=intersec2topos)
            newPosDesiredx = PosDesiredx;
            newPosDesiredy = PosDesiredy;
            zerochk = 0;
            wperpendicular = (w + 0.5 * pi)*zerochk;
        elseif(desiredtopos<=intersec1topos && desiredtopos>intersec2topos)
            newPosDesiredx = intersectx2;
            newPosDesiredy = intersecty2;
            zerochk = 0;
            wperpendicular = (w + 0.5 * pi)*zerochk;
        elseif(desiredtopos>intersec1topos && desiredtopos<=intersec2topos)  
            newPosDesiredx = intersectx1;
            newPosDesiredy = intersecty1;
            zerochk = 0;
            wperpendicular = (w + 0.5 * pi)*zerochk;
        else
            zerochk = 1;
            wperpendicular = (w + 0.5 * pi)*zerochk;
            if(intersec1topos<intersec2topos)
            newPosDesiredx = 0.5*cos(wperpendicular) + intersectx1;
            newPosDesiredy = 0.5*sin(wperpendicular) + intersecty1;
            else
            newPosDesiredx = 0.5*cos(wperpendicular) + intersectx2;
            newPosDesiredy = 0.5*sin(wperpendicular) + intersecty2;  
            end
            
        end
    
end 
end

== matlab function Car_22_Jan_test_2012b/UAV 1/Trajectory Logic/matchcontrol ==
  data: match_flag output; posx input; posy input; Cpx input; Cpy input
function match_flag  = fcn(posx,posy,Cpx,Cpy)
%#codegen
if(abs(Cpx-posx)+abs(Cpy-posy)<0.3)
    match_flag = 1;
else
    match_flag = 0;
end

== matlab function Car_22_Jan_test_2012b/UAV 1/Trajectory Logic/masscontrol1 ==
  data: mass output; Cpz input; capture output
function [mass,capture]  = fcn(Cpz)
%#codegen

if( Cpz <-0.1)%match_flag==1 && Cpz<=-0.07 &&
    mass = 1.2;
    capture = 0;
else
    mass = 0.84;
    capture = 1;
    
end

== matlab function Car_22_Jan_test_2012b/UAV 1/Trajectory Logic/MATLAB Function ==
  data: smooth_flag input; bfboundx input; finalx output; finaly output; bfboundy input
function [finalx,finaly] = fcn(smooth_flag,bfboundx,bfboundy)
%#codegen
if(smooth_flag == 1)
    finalx = bfboundx;
    finaly = bfboundy;
else
    if(bfboundx >= 2.489)
        finalx = 2.489;
    elseif(bfboundx <= -2.83)
        finalx = -2.83;
    else
        finalx = bfboundx;
    end
     if(bfboundy >= 3)
        finaly = 3;
    elseif(bfboundy <= -2.345)
        finaly = -2.345;
    else
        finaly = bfboundy;
     end
end

== matlab function Car_22_Jan_test_2012b/UAV 1/Trajectory Logic/timercontrol ==
  data: zero input; y output; timeenable input; capture input
function y = fcn(zero,timeenable,capture)
%#codegen
if(zero == 0||capture ==0||timeenable==0)
    y = 0;
else
   y = 1; 
end

== stateflow chart Car_22_Jan_test_2012b/UAV 1/Trajectory Logic/stateflowforwholesequence ==
  state Airborne1
    state capturing_sequence
      state caputuring_test1
        en: PosDesired = Pos; PosDesired[2] = -1.2;smooth_flag = 1;timerenable = 0;
      state capturing_sequence1
        state capturing_sequence2
          state normal_capturing1
            en: PosDesired[0] = carest[0] ; PosDesired[1] = carest[1] ; PosDesired[2] = -0.5;pwm = 1650;
          state normal_capturing3
            du: PosDesired[0] = car[0] ; PosDesired[1] = car[1]; PosDesired[2] = -0.5;pwm = 1250;
          state normal_capturing2
            du: PosDesired[0] = car[0] ; PosDesired[1] = car[1]; PosDesired[2] = -0.5;pwm = 1250;
          state match_chk
            state caputuring_test1
              en:PosDesired = Pos;PosDesired[2] = -1.2;
            state caputuring_test2
              en: PosDesired[0] = 0.15*(0-car[0])/abs(0-car[0]);
              PosDesired[1] = 0.15*(0-car[1])/abs(0-car[1]);
            state caputuring_test
              en: PosDesired[2] = -0.5;
            (default) -> (junction 60) : {PosDesired = Pos;pwm = 1450;PosDesired[2] = -1.2}
            (junction 60) -> Airborne1.capturing_sequence.capturing_sequence1.capturing_sequence2.match_chk.caputuring_test1 [order 1] : [abs(Pos[2]-car[2])<0.5]
            (junction 60) -> caputuring_test [order 2] : [abs(Pos[2]-car[2])>0.5]
            caputuring_test2 -> Airborne1.capturing_sequence.capturing_sequence1.capturing_sequence2.match_chk.caputuring_test1 : after(2,sec)
            caputuring_test -> caputuring_test2 : [abs(Pos[2]+0.5)<0.1]
          (junction 105) -> normal_capturing3 [order 1] : [(directionflag == 0)||(directionflag==-1)]
          (default) -> (junction 105)
          (junction 105) -> normal_capturing1 [order 2] : [directionflag == 1]
          normal_capturing3 -> normal_capturing1 : [directionflag == 1]
          normal_capturing2 -> normal_capturing1 [order 2] : [(frontbackflag == 0)&&(match_flag ~=1)]
          normal_capturing1 -> normal_capturing2 [order 2] : [((abs(carest[0] - Pos[0])+abs(carest[1] - Pos[1]))<0.15)&&(match_flag~=1)]
          normal_capturing1 -> match_chk [order 1] : after(1,sec)
              | [match_flag==1]
          normal_capturing2 -> match_chk [order 1] : after(1,sec)
              | [match_flag==1]
          match_chk -> normal_capturing2 : [match_flag~=1]
        state Hover2
          en: PosDesired[2] = -1.2;
        (default) -> Hover2 : {PosDesired = Pos;smooth_flag = 0;pwm = 2100;timerenable = 1;}
        Hover2 -> capturing_sequence2 : after(3,sec)
      state move_origin7
        du:PosDesired[1] = (0 - PosDesired[1])*0.5*DeltaT + PosDesired[1] ;
        PosDesired[0] = (0 - PosDesired[0])*0.7*DeltaT + PosDesired[0] ;
        PosDesired[2] = -1.2;
      state move_origin6
        du:PosDesired[0] = 0;
        PosDesired[1] = (ly - PosDesired[1])*0.5*DeltaT + PosDesired[1] ;
        PosDesired[2] = -1.2;
      state move_origin5
        du:PosDesired[0] = (lx - PosDesired[0])*0.5*DeltaT + PosDesired[0] ;
        PosDesired[1] = ly;
        PosDesired[2] = -1.2;
      state hoverstate
        en:PosDesired = Pos;PosDesired[2] = -1.2;pwm = 1450;
      capturing_sequence1 -> Airborne1.capturing_sequence.caputuring_test1 [order 1] : after(93,sec)
      (default) -> capturing_sequence1
      capturing_sequence1 -> Airborne1.capturing_sequence.caputuring_test1 [order 3] : [RC[5] < 0]
      capturing_sequence1 -> Airborne1.capturing_sequence.caputuring_test1 [order 2] : [car[2]<-0.4]
      Airborne1.capturing_sequence.caputuring_test1 -> (junction 61) : [abs(Pos[2]+1.2)<0.2]
      (junction 61) -> move_origin7 [order 1] : [car[2]>-0.4]
          | {pwm = 1350;}
      (junction 61) -> move_origin7 [order 3] : [RC[5]<0]
          | {pwm = 2100;}
      (junction 61) -> move_origin7 [order 2] : [car[2]<-0.4]
          | {pwm = 1550;}
      move_origin7 -> move_origin6 : [(abs(0 - Pos[0])+abs(0 - Pos[1]))<0.15]
      move_origin6 -> move_origin5 : [(abs(0 - Pos[0])+abs(ly-Pos[1]))<0.1]
      move_origin5 -> hoverstate : [(abs(lx - Pos[0])+abs(ly - Pos[1]))<0.1]
    state TakeOff
      du:HoverThrottle = (H0 - HoverThrottle)*2*DeltaT + HoverThrottle ;
    state Hover
      en: PosDesired[2] = -1.2;
    state move_origin
      du:PosDesired[0] = (0 - PosDesired[0])*1*DeltaT + PosDesired[0] ;PosDesired[1] = ly;
      PosDesired[2] = -1.2;
    state move_origin1
      du:PosDesired[1] = (0 - PosDesired[1])*1*DeltaT + PosDesired[1] ;PosDesired[0] = 0;
      PosDesired[2] = -1.2;
    state Hover1
      en: PosDesired[2] = -1.2;pwm = 1450;
    (default) -> TakeOff : {PosDesired = Pos;PosDesired[2] = -1.2;lx = Pos[0];ly = Pos[1];lz = Pos[2];smooth_flag = 1;pwm = 1650;timerenable = 0;}
    TakeOff -> Hover : after(3,sec)
    Hover -> move_origin : after(5,sec)
    move_origin -> move_origin1 : after(5,sec)
    move_origin1 -> Hover1 : [(abs(0 - Pos[0])+abs(0 - Pos[1]))<0.2]
        | {PosDesired = Pos;}
    Hover1 -> capturing_sequence : [RC[5] > 0]
        | {relay = 1;}
  state Landing
    state Decsending
      en:smooth_flag = 1;pwm = 1850;
      du:PosDesired[2] = (lz - PosDesired[2])*0.7*DeltaT + PosDesired[2] ;
    state CutThrottle
      du:HoverThrottle = (0.0 - HoverThrottle)*2*DeltaT + HoverThrottle ;
    (default) -> Decsending : {PosDesired = Pos;smooth_flag = 1;}
    Decsending -> CutThrottle : [Pos[2] > lz-0.15]
  Landing -> Airborne1 : [RC[6] > 0.5]
  Airborne1 -> Landing : [RC[6] < -0.5]
  (default) -> Landing : {HoverThrottle=0.01;}
  data: PosDesired output double size=4; HoverThrottle output double size=1; RC input size=8; Pos input size=4; DeltaT parameter size=1; H0 parameter size=1; Kl parameter size=1; VelCmd local double size=2 =0; line_count local int8 size=1 =0; triangle_count local int8 size=1 =0; T_line local double size=1; omega_circle parameter size=1; PI parameter size=1; omega_h parameter; Circle_R parameter size=1; MAX_Height parameter size=1; car input size=12; carest input size=2; match_flag input; smooth_flag output boolean =0; matchx local double; matchy local double; pwm output; lx local double; ly local double; pwm1 local double; relay output; timerenable output; lz local double; laflag local boolean; directionflag input; frontbackflag input

== matlab function Car_22_Jan_test_2012b/UAV 1/Vertical Controller/MATLAB Function ==
  data: u input; y output
function y = fcn(u)
%#codegen
if u > 0.5;
    y = 0;
else 
    y = 1;
end
